simulink model "ModeInt"  (R2018b)
settings: Solver=FixedStepDiscrete  StartTime=0.0  StopTime=10.0  FixedStep=0.01  RelTol=1e-3
undefined symbols (not defined in the file or in its folder): c, CmprtMdHMIReqTp1, e, IfVeSMSeStNumConfig, MdReqTp1
(part 1 of 4)
settings Model: Creator=su3dcu  LastModifiedBy=su3dcu
settings DataIOCC: SaveFormat=StructureWithTime  ReturnWorkspaceOutputs=on
settings OptimizationCC: DefaultParameterBehavior=Inlined  EnhancedBackFolding=on  PassReuseOutputArgsAs=Individual arguments  ZeroExternalMemoryAtStartup=off  ZeroInternalMemoryAtStartup=off  OptimizeBlockOrder=speed  DifferentSizesBufferReuse=on  OptimizationCustomize=off
settings DebuggingCC: ParameterTunabilityLossMsg=error
settings HardwareCC: ProdBitPerPointer=32  ProdBitPerSizeT=32  ProdBitPerPtrDiffT=32  ProdLargestAtomicFloat=None  ProdWordSize=32  ProdHWDeviceType=Renesas->RH850
settings ModelReferenceCC: ModelReferenceNumInstancesAllowed=Single
settings SFSimCC: SimCustomHeaderCode="#include\"Rte_Type.h\""  MATLABDynamicMemAlloc=off
settings RTWCC: SystemTargetFile=autosar.tlc  GenCodeOnly=on  TemplateMakefile=ert_default_tmf  Description=AUTOSAR  GenerateReport=on  IncludeHyperlinkInReport=on  LaunchReport=on  CodeExecutionProfiling=on  GenerateTraceInfo=on  GenerateTraceReport=on  GenerateTraceReportSl=on  GenerateTraceReportSf=on  GenerateTraceReportEml=on  GenerateCodeMetricsReport=on
settings CodeAppCC: ForceParamTrailComments=on  IgnoreCustomStorageClasses=off  MaxIdLength=63  OperatorAnnotations=on  SimulinkDataObjDesc=on  SFDataObjDesc=on  InsertBlockDesc=on
settings STFCustomTargetCC: TargetLangStandard=C99 (ISO)  MultiwordLength=256  ParMdlRefBuildCompliant=on  CompOptLevelCompliant=on  IncludeMdlTerminateFcn=off  CombineOutputUpdateFcns=on  SuppressErrorStatus=on  ERTCustomFileBanners=on  SupportAbsoluteTime=off  PurelyIntegerCode=on  SupportNonFinite=off  SupportComplex=off  SupportContinuousTime=off  SupportNonInlinedSFcns=off  RemoveResetFunc=on  MATLABClassNameForMDSCustomization=Simulink.SoftwareTarget.ERTCustomization  AutosarCompliant=on  UseToolchainInfoCompliant=on  LookupTableObjectStructAxisOrder=2,1,3,4,...  LUTObjectStructOrderEvenSpacing=Size,Table,Breakpoints  SystemTargetFile=autosar.tlc
settings ERTTargetCC: TargetLangStandard=C99 (ISO)  ConcurrentExecutionCompliant=off  IncludeMdlTerminateFcn=off  SuppressErrorStatus=on  SupportAbsoluteTime=off  PurelyIntegerCode=on  SupportNonFinite=off  SupportComplex=off  ModelStepFunctionPrototypeControlCompliant=off  CPPClassGenCompliant=off  AutosarCompliant=on  LookupTableObjectStructAxisOrder=2,1,3,4,...  LUTObjectStructOrderEvenSpacing=Size,Table,Breakpoints  InlinedParameterPlacement=NonHierarchical  ERTCustomFileTemplate=example_file_process.tlc  ERTFilePackagingFormat=Compact
settings ConfigComp: DVTestSuiteOptimization=CombinedObjectives (Nonlinear Extended)  DVDetectActiveLogic=on  DVDetectOutOfBounds=on

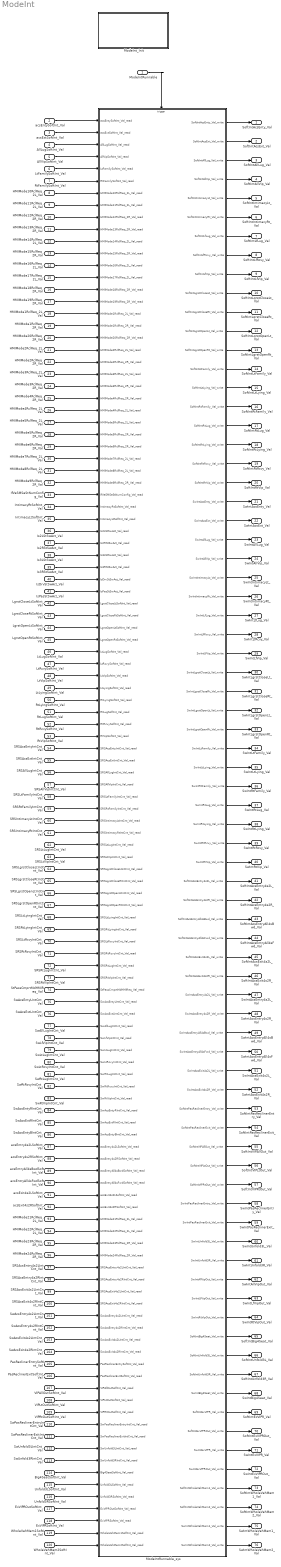
== system ModeInt ==
  ModeIntRunnable : Inport  SampleTime=0.01  OutputFunctionCall=on
  acsEntySoftInt_Val : Inport  Port=2  OutDataTypeStr=IntEnable  PortDimensions=1
  acsExtSoftInt_Val : Inport  Port=3  OutDataTypeStr=IntEnable  PortDimensions=1
  AllLugSoftInt_Val : Inport  Port=4  OutDataTypeStr=IntEnable  PortDimensions=1
  AllVipSoftInt_Val : Inport  Port=5  OutDataTypeStr=IntEnable  PortDimensions=1
  LtFamilySoftInt_Val : Inport  Port=6  OutDataTypeStr=IntEnable  PortDimensions=1
  RtFamilySoftInt_Val : Inport  Port=7  OutDataTypeStr=IntEnable  PortDimensions=1
  HMIMode10RclReq_2L_Val : Inport  Port=8  OutDataTypeStr=Enum: MdReqTp1  PortDimensions=1
  HMIMode11RclReq_2L_Val : Inport  Port=9  OutDataTypeStr=Enum: MdReqTp1  PortDimensions=1
  HMIMode12RclReq_2R_Val : Inport  Port=10  OutDataTypeStr=Enum: MdReqTp1  PortDimensions=1
  HMIMode13RclReq_2R_Val : Inport  Port=11  OutDataTypeStr=Enum: MdReqTp1  PortDimensions=1
  HMIMode14RclReq_2L_Val : Inport  Port=12  OutDataTypeStr=Enum: MdReqTp1  PortDimensions=1
  HMIMode15RclReq_2R_Val : Inport  Port=13  OutDataTypeStr=Enum: MdReqTp1  PortDimensions=1
  HMIMode16RclReq_2L_Val : Inport  Port=14  OutDataTypeStr=Enum: MdReqTp1  PortDimensions=1
  HMIMode17RclReq_2L_Val : Inport  Port=15  OutDataTypeStr=Enum: MdReqTp1  PortDimensions=1
  HMIMode18RclReq_2R_Val : Inport  Port=16  OutDataTypeStr=Enum: MdReqTp1  PortDimensions=1
  HMIMode19RclReq_2R_Val : Inport  Port=17  OutDataTypeStr=Enum: MdReqTp1  PortDimensions=1
  HMIMode1RclReq_2L_Val : Inport  Port=18  OutDataTypeStr=Enum: MdReqTp1  PortDimensions=1
  HMIMode1RclReq_2R_Val : Inport  Port=19  OutDataTypeStr=Enum: MdReqTp1  PortDimensions=1
  HMIMode20RclReq_2R_Val : Inport  Port=20  OutDataTypeStr=Enum: MdReqTp1  PortDimensions=1
  HMIMode2RclReq_2L_Val : Inport  Port=21  OutDataTypeStr=Enum: MdReqTp1  PortDimensions=1
  HMIMode2RclReq_2R_Val : Inport  Port=22  OutDataTypeStr=Enum: MdReqTp1  PortDimensions=1
  HMIMode3RclReq_2L_Val : Inport  Port=23  OutDataTypeStr=Enum: MdReqTp1  PortDimensions=1
  HMIMode3RclReq_2R_Val : Inport  Port=24  OutDataTypeStr=Enum: MdReqTp1  PortDimensions=1
  HMIMode4RclReq_2R_Val : Inport  Port=25  OutDataTypeStr=Enum: MdReqTp1  PortDimensions=1
  HMIMode4RclReq_2L_Val : Inport  Port=26  OutDataTypeStr=Enum: MdReqTp1  PortDimensions=1
  HMIMode5RclReq_2L_Val : Inport  Port=27  OutDataTypeStr=Enum: MdReqTp1  PortDimensions=1
  HMIMode5RclReq_2R_Val : Inport  Port=28  OutDataTypeStr=Enum: MdReqTp1  PortDimensions=1
  HMIMode6RclReq_2R_Val : Inport  Port=29  OutDataTypeStr=Enum: MdReqTp1  PortDimensions=1
  HMIMode7RclReq_2L_Val : Inport  Port=30  OutDataTypeStr=Enum: MdReqTp1  PortDimensions=1
  HMIMode8RclReq_2L_Val : Inport  Port=31  OutDataTypeStr=Enum: MdReqTp1  PortDimensions=1
  HMIMode9RclReq_2R_Val : Inport  Port=32  OutDataTypeStr=Enum: MdReqTp1  PortDimensions=1
  IfVeSMSeStNumConfig_Val : Inport  Port=33  OutDataTypeStr=Enum: IfVeSMSeStNumConfig  PortDimensions=1
  IntimacyRtSoftInt_Val : Inport  Port=34  OutDataTypeStr=IntEnable  PortDimensions=1
  IntimacyLtSoftInt_Val : Inport  Port=35  OutDataTypeStr=IntEnable  PortDimensions=1
  Is2LStSwAct_Val : Inport  Port=36  OutDataTypeStr=boolean  PortDimensions=1
  Is2RStSwAct_Val : Inport  Port=37  OutDataTypeStr=boolean  PortDimensions=1
  Is3LStSwAct_Val : Inport  Port=38  OutDataTypeStr=boolean  PortDimensions=1
  Is3RStSwAct_Val : Inport  Port=39  OutDataTypeStr=boolean  PortDimensions=1
  IsDrvStSwAct_Val : Inport  Port=40  OutDataTypeStr=boolean  PortDimensions=1
  IsPasStSwAct_Val : Inport  Port=41  OutDataTypeStr=boolean  PortDimensions=1
  LgrstCloseLtSoftInt_Val : Inport  Port=42  OutDataTypeStr=IntEnable  PortDimensions=1
  LgrstCloseRtSoftInt_Val : Inport  Port=43  OutDataTypeStr=IntEnable  PortDimensions=1
  LgrstOpenLtSoftInt_Val : Inport  Port=44  OutDataTypeStr=IntEnable  PortDimensions=1
  LgrstOpenRtSoftInt_Val : Inport  Port=45  OutDataTypeStr=IntEnable  PortDimensions=1
  LtLugSoftInt_Val : Inport  Port=46  OutDataTypeStr=IntEnable  PortDimensions=1
  LtRcvySoftInt_Val : Inport  Port=47  OutDataTypeStr=IntEnable  PortDimensions=1
  LtVipSoftInt_Val : Inport  Port=48  OutDataTypeStr=IntEnable  PortDimensions=1
  LtLyingSoftInt_Val : Inport  Port=49  OutDataTypeStr=IntEnable  PortDimensions=1
  RtLyingSoftInt_Val : Inport  Port=50  OutDataTypeStr=IntEnable  PortDimensions=1
  RtLugSoftInt_Val : Inport  Port=51  OutDataTypeStr=IntEnable  PortDimensions=1
  RtRcvySoftInt_Val : Inport  Port=52  OutDataTypeStr=IntEnable  PortDimensions=1
  RtVipSoftInt_Val : Inport  Port=53  OutDataTypeStr=IntEnable  PortDimensions=1
  SRSAcsEntyIntCnt_Val : Inport  Port=54  OutDataTypeStr=IntCnt  PortDimensions=1
  SRSAcsExtIntCnt_Val : Inport  Port=55  OutDataTypeStr=IntCnt  PortDimensions=1
  SRSAllLugIntCnt_Val : Inport  Port=56  OutDataTypeStr=IntCnt  PortDimensions=1
  SRSAllVipIntCnt_Val : Inport  Port=57  OutDataTypeStr=IntCnt  PortDimensions=1
  SRSLtFamilyIntCnt_Val : Inport  Port=58  OutDataTypeStr=IntCnt  PortDimensions=1
  SRSRtFamilyIntCnt_Val : Inport  Port=59  OutDataTypeStr=IntCnt  PortDimensions=1
  SRSIntimacyLtIntCnt_Val : Inport  Port=60  OutDataTypeStr=IntCnt  PortDimensions=1
  SRSIntimacyRtIntCnt_Val : Inport  Port=61  OutDataTypeStr=IntCnt  PortDimensions=1
  SRSLtLugIntCnt_Val : Inport  Port=62  OutDataTypeStr=IntCnt  PortDimensions=1
  SRSLtVipIntCnt_Val : Inport  Port=63  OutDataTypeStr=IntCnt  PortDimensions=1
  SRSLgrstCloseLtIntCnt_Val : Inport  Port=64  OutDataTypeStr=IntCnt  PortDimensions=1
  SRSLgrstCloseRtIntCnt_Val : Inport  Port=65  OutDataTypeStr=IntCnt  PortDimensions=1
  SRSLgrstOpenLtIntCnt_Val : Inport  Port=66  OutDataTypeStr=IntCnt  PortDimensions=1
  SRSLgrstOpenRtIntCnt_Val : Inport  Port=67  OutDataTypeStr=IntCnt  PortDimensions=1
  SRSLtLyingIntCnt_Val : Inport  Port=68  OutDataTypeStr=IntCnt  PortDimensions=1
  SRSRtLyingIntCnt_Val : Inport  Port=69  OutDataTypeStr=IntCnt  PortDimensions=1
  SRSLtRcvyIntCnt_Val : Inport  Port=70  OutDataTypeStr=IntCnt  PortDimensions=1
  SRSRtRcvyIntCnt_Val : Inport  Port=71  OutDataTypeStr=IntCnt  PortDimensions=1
  SRSRtLugIntCnt_Val : Inport  Port=72  OutDataTypeStr=IntCnt  PortDimensions=1
  SRSRtVipIntCnt_Val : Inport  Port=73  OutDataTypeStr=IntCnt  PortDimensions=1
  StPassCmprtMdHMIReq_Val : Inport  Port=74  OutDataTypeStr=Enum: CmprtMdHMIReqTp1  PortDimensions=1
  SwAcsEntyLIntCnt_Val : Inport  Port=75  OutDataTypeStr=IntCnt  PortDimensions=1
  SwAcsExtLIntCnt_Val : Inport  Port=76  OutDataTypeStr=IntCnt  PortDimensions=1
  SwAllLugIntCnt_Val : Inport  Port=77  OutDataTypeStr=IntCnt  PortDimensions=1
  SwLfVipIntCnt_Val : Inport  Port=78  OutDataTypeStr=IntCnt  PortDimensions=1
  SwLtLugIntCnt_Val : Inport  Port=79  OutDataTypeStr=IntCnt  PortDimensions=1
  SwLtRcvyIntCnt_Val : Inport  Port=80  OutDataTypeStr=IntCnt  PortDimensions=1
  SwRtLugIntCnt_Val : Inport  Port=81  OutDataTypeStr=IntCnt  PortDimensions=1
  SwRtRcvyIntCnt_Val : Inport  Port=82  OutDataTypeStr=IntCnt  PortDimensions=1
  SwRtVipIntCnt_Val : Inport  Port=83  OutDataTypeStr=IntCnt  PortDimensions=1
  SwAcsEntyRIntCnt_Val : Inport  Port=84  OutDataTypeStr=IntCnt  PortDimensions=1
  SwAcsExtRIntCnt_Val : Inport  Port=85  OutDataTypeStr=IntCnt  PortDimensions=1
  SwAcsEntyBIntCnt_Val : Inport  Port=86  OutDataTypeStr=IntCnt  PortDimensions=1
  acsEntry4s2LSoftInt_Val : Inport  Port=87  OutDataTypeStr=IntEnable  PortDimensions=1
  acsEntry4s2RSoftInt_Val : Inport  Port=88  OutDataTypeStr=IntEnable  PortDimensions=1
  acsEntryAll4sBwdSoftInt_Val : Inport  Port=89  OutDataTypeStr=IntEnable  PortDimensions=1
  acsEntryAll4sFwdSoftInt_Val : Inport  Port=90  OutDataTypeStr=IntEnable  PortDimensions=1
  acsExit4s2LSoftInt_Val : Inport  Port=91  OutDataTypeStr=IntEnable  PortDimensions=1
  acsExit4s2RSoftInt_Val : Inport  Port=92  OutDataTypeStr=IntEnable  PortDimensions=1
  HMIMode21RclReq_2L_Val : Inport  Port=93  OutDataTypeStr=Enum: MdReqTp1  PortDimensions=1
  HMIMode22RclReq_2L_Val : Inport  Port=94  OutDataTypeStr=Enum: MdReqTp1  PortDimensions=1
  HMIMode23RclReq_2R_Val : Inport  Port=95  OutDataTypeStr=Enum: MdReqTp1  PortDimensions=1
  HMIMode24RclReq_2R_Val : Inport  Port=96  OutDataTypeStr=Enum: MdReqTp1  PortDimensions=1
  SRSAcsEntry4s2LIntCnt_Val : Inport  Port=97  OutDataTypeStr=IntCnt  PortDimensions=1
  SRSAcsEntry4s2RIntCnt_Val : Inport  Port=98  OutDataTypeStr=IntCnt  PortDimensions=1
  SRSAcsExit4s2LIntCnt_Val : Inport  Port=99  OutDataTypeStr=IntCnt  PortDimensions=1
  SRSAcsExit4s2RIntCnt_Val : Inport  Port=100  OutDataTypeStr=IntCnt  PortDimensions=1
  SwAcsEntry4s2LIntCnt_Val : Inport  Port=101  OutDataTypeStr=IntCnt  PortDimensions=1
  SwAcsEntry4s2RIntCnt_Val : Inport  Port=102  OutDataTypeStr=IntCnt  PortDimensions=1
  SwAcsExit4s2LIntCnt_Val : Inport  Port=103  OutDataTypeStr=IntCnt  PortDimensions=1
  SwAcsExit4s2RIntCnt_Val : Inport  Port=104  OutDataTypeStr=IntCnt  PortDimensions=1
  PasReclinerEntrySoftInt_Val : Inport  Port=105  OutDataTypeStr=IntEnable  PortDimensions=1
  PasReclinerExitSoftInt_Val : Inport  Port=106  OutDataTypeStr=IntEnable  PortDimensions=1
  VIPAllOutSoftInt_Val : Inport  Port=107  OutDataTypeStr=IntEnable  PortDimensions=1
  VIPLtOutSoftInt_Val : Inport  Port=108  OutDataTypeStr=IntEnable  PortDimensions=1
  VIPRtOutSoftInt_Val : Inport  Port=109  OutDataTypeStr=IntEnable  PortDimensions=1
  SwPasReclinerEntryIntCnt_Val : Inport  Port=110  OutDataTypeStr=IntCnt  PortDimensions=1
  SwPasReclinerExitIntCnt_Val : Inport  Port=111  OutDataTypeStr=IntCnt  PortDimensions=1
  SwUnfold3LIntCnt_Val : Inport  Port=112  OutDataTypeStr=IntCnt  PortDimensions=1
  SwUnfold3RIntCnt_Val : Inport  Port=113  OutDataTypeStr=IntCnt  PortDimensions=1
  Big4SeatSoftInt_Val : Inport  Port=114  OutDataTypeStr=IntEnable  PortDimensions=1
  Unfold3LSoftInt_Val : Inport  Port=115  OutDataTypeStr=IntEnable  PortDimensions=1
  Unfold3RSoftInt_Val : Inport  Port=116  OutDataTypeStr=IntEnable  PortDimensions=1
  ExVIPROutSoftInt_Val : Inport  Port=117  OutDataTypeStr=IntEnable  PortDimensions=1
  ExVIPRSoftInt_Val : Inport  Port=118  OutDataTypeStr=IntEnable  PortDimensions=1
  WholeVehMem1SoftInt_Val : Inport  Port=119  OutDataTypeStr=IntEnable  PortDimensions=1
  WholeVehMem2SoftInt_Val : Inport  Port=120  OutDataTypeStr=IntEnable  PortDimensions=1
  ModeIntRunnable_sys : Subsystem
  ModeInt_Init : Subsystem
  SoftIntAcsEnty_Val : Outport  OutDataTypeStr=IntEnable  PortDimensions=1
  SoftIntAcsExt_Val : Outport  Port=2  OutDataTypeStr=IntEnable  PortDimensions=1
  SoftIntAllLug_Val : Outport  Port=3  OutDataTypeStr=IntEnable  PortDimensions=1
  SoftIntAllVip_Val : Outport  Port=4  OutDataTypeStr=IntEnable  PortDimensions=1
  SoftIntIntimacyLt_Val : Outport  Port=5  OutDataTypeStr=IntEnable  PortDimensions=1
  SoftIntIntimacyRt_Val : Outport  Port=6  OutDataTypeStr=IntEnable  PortDimensions=1
  SoftIntLfLug_Val : Outport  Port=7  OutDataTypeStr=IntEnable  PortDimensions=1
  SoftIntLfRcvy_Val : Outport  Port=8  OutDataTypeStr=IntEnable  PortDimensions=1
  SoftIntLfVip_Val : Outport  Port=9  OutDataTypeStr=IntEnable  PortDimensions=1
  SoftIntLgrstCloseLt_Val : Outport  Port=10  OutDataTypeStr=IntEnable  PortDimensions=1
  SoftIntLgrstCloseRt_Val : Outport  Port=11  OutDataTypeStr=IntEnable  PortDimensions=1
  SoftIntLgrstOpenLt_Val : Outport  Port=12  OutDataTypeStr=IntEnable  PortDimensions=1
  SoftIntLgrstOpenRt_Val : Outport  Port=13  OutDataTypeStr=IntEnable  PortDimensions=1
  SoftIntLtFamily_Val : Outport  Port=14  OutDataTypeStr=IntEnable  PortDimensions=1
  SoftIntLtLying_Val : Outport  Port=15  OutDataTypeStr=IntEnable  PortDimensions=1
  SoftIntRtFamily_Val : Outport  Port=16  OutDataTypeStr=IntEnable  PortDimensions=1
  SoftIntRtLug_Val : Outport  Port=17  OutDataTypeStr=IntEnable  PortDimensions=1
  SoftIntRtLying_Val : Outport  Port=18  OutDataTypeStr=IntEnable  PortDimensions=1
  SoftIntRtRcvy_Val : Outport  Port=19  OutDataTypeStr=IntEnable  PortDimensions=1
  SoftIntRtVip_Val : Outport  Port=20  OutDataTypeStr=IntEnable  PortDimensions=1
  SwIntAcsEnty_Val : Outport  Port=21  OutDataTypeStr=IntEnable  PortDimensions=1
  SwIntAcsExt_Val : Outport  Port=22  OutDataTypeStr=IntEnable  PortDimensions=1
  SwIntAllLug_Val : Outport  Port=23  OutDataTypeStr=IntEnable  PortDimensions=1
  SwIntAllVip_Val : Outport  Port=24  OutDataTypeStr=IntEnable  PortDimensions=1
  SwIntIntimacyLt_Val : Outport  Port=25  OutDataTypeStr=IntEnable  PortDimensions=1
  SwIntIntimacyRt_Val : Outport  Port=26  OutDataTypeStr=IntEnable  PortDimensions=1
  SwIntLfLug_Val : Outport  Port=27  OutDataTypeStr=IntEnable  PortDimensions=1
  SwIntLfRcvy_Val : Outport  Port=28  OutDataTypeStr=IntEnable  PortDimensions=1
  SwIntLfVip_Val : Outport  Port=29  OutDataTypeStr=IntEnable  PortDimensions=1
  SwIntLgrstCloseLt_Val : Outport  Port=30  OutDataTypeStr=IntEnable  PortDimensions=1
  SwIntLgrstCloseRt_Val : Outport  Port=31  OutDataTypeStr=IntEnable  PortDimensions=1
  SwIntLgrstOpenLt_Val : Outport  Port=32  OutDataTypeStr=IntEnable  PortDimensions=1
  SwIntLgrstOpenRt_Val : Outport  Port=33  OutDataTypeStr=IntEnable  PortDimensions=1
  SwIntLtFamily_Val : Outport  Port=34  OutDataTypeStr=IntEnable  PortDimensions=1
  SwIntLtLying_Val : Outport  Port=35  OutDataTypeStr=IntEnable  PortDimensions=1
  SwIntRtFamily_Val : Outport  Port=36  OutDataTypeStr=IntEnable  PortDimensions=1
  SwIntRtLug_Val : Outport  Port=37  OutDataTypeStr=IntEnable  PortDimensions=1
  SwIntRtLying_Val : Outport  Port=38  OutDataTypeStr=IntEnable  PortDimensions=1
  SwIntRtRcvy_Val : Outport  Port=39  OutDataTypeStr=IntEnable  PortDimensions=1
  SwIntRtVip_Val : Outport  Port=40  OutDataTypeStr=IntEnable  PortDimensions=1
  SoftIntAcsEntry4s2L_Val : Outport  Port=41  OutDataTypeStr=IntEnable  PortDimensions=1
  SoftIntAcsEntry4s2R_Val : Outport  Port=42  OutDataTypeStr=IntEnable  PortDimensions=1
  SoftIntAcsEntryAll4sBwd_Val : Outport  Port=43  OutDataTypeStr=IntEnable  PortDimensions=1
  SoftIntAcsEntryAll4sFwd_Val : Outport  Port=44  OutDataTypeStr=IntEnable  PortDimensions=1
  SoftIntAcsExit4s2L_Val : Outport  Port=45  OutDataTypeStr=IntEnable  PortDimensions=1
  SoftIntAcsExit4s2R_Val : Outport  Port=46  OutDataTypeStr=IntEnable  PortDimensions=1
  SwIntAcsEntry4s2L_Val : Outport  Port=47  OutDataTypeStr=IntEnable  PortDimensions=1
  SwIntAcsEntry4s2R_Val : Outport  Port=48  OutDataTypeStr=IntEnable  PortDimensions=1
  SwIntAcsEntryAll4sBwd_Val : Outport  Port=49  OutDataTypeStr=IntEnable  PortDimensions=1
  SwIntAcsEntryAll4sFwd_Val : Outport  Port=50  OutDataTypeStr=IntEnable  PortDimensions=1
  SwIntAcsExit4s2L_Val : Outport  Port=51  OutDataTypeStr=IntEnable  PortDimensions=1
  SwIntAcsExit4s2R_Val : Outport  Port=52  OutDataTypeStr=IntEnable  PortDimensions=1
  SoftIntPasReclinerEntry_Val : Outport  Port=53  OutDataTypeStr=IntEnable  PortDimensions=1
  SoftIntPasReclinerExit_Val : Outport  Port=54  OutDataTypeStr=IntEnable  PortDimensions=1
  SoftIntVIPAllOut_Val : Outport  Port=55  OutDataTypeStr=IntEnable  PortDimensions=1
  SoftIntVIPLtOut_Val : Outport  Port=56  OutDataTypeStr=IntEnable  PortDimensions=1
  SoftIntVIPRtOut_Val : Outport  Port=57  OutDataTypeStr=IntEnable  PortDimensions=1
  SwIntPasReclinerEntry_Val : Outport  Port=58  OutDataTypeStr=IntEnable  PortDimensions=1
  SwIntPasReclinerExit_Val : Outport  Port=59  OutDataTypeStr=IntEnable  PortDimensions=1
  SwIntUnfold3L_Val : Outport  Port=60  OutDataTypeStr=IntEnable  PortDimensions=1
  SwIntUnfold3R_Val : Outport  Port=61  OutDataTypeStr=IntEnable  PortDimensions=1
  SwIntAllVipOut_Val : Outport  Port=62  OutDataTypeStr=IntEnable  PortDimensions=1
  SwIntLfVipOut_Val : Outport  Port=63  OutDataTypeStr=IntEnable  PortDimensions=1
  SwIntRtVipOut_Val : Outport  Port=64  OutDataTypeStr=IntEnable  PortDimensions=1
  SoftIntBig4Seat_Val : Outport  Port=65  OutDataTypeStr=IntEnable  PortDimensions=1
  SoftIntUnfold3L_Val : Outport  Port=66  OutDataTypeStr=IntEnable  PortDimensions=1
  SoftIntUnfold3R_Val : Outport  Port=67  OutDataTypeStr=IntEnable  PortDimensions=1
  SwIntBig4Seat_Val : Outport  Port=68  OutDataTypeStr=IntEnable  PortDimensions=1
  SoftIntExVIPR_Val : Outport  Port=69  OutDataTypeStr=IntEnable  PortDimensions=1
  SoftIntExVIPROut_Val : Outport  Port=70  OutDataTypeStr=IntEnable  PortDimensions=1
  SwIntExVIPR_Val : Outport  Port=71  OutDataTypeStr=IntEnable  PortDimensions=1
  SwIntExVIPROut_Val : Outport  Port=72  OutDataTypeStr=IntEnable  PortDimensions=1
  SoftIntWholeVehMem1_Val : Outport  Port=73  OutDataTypeStr=IntEnable  PortDimensions=1
  SoftIntWholeVehMem2_Val : Outport  Port=74  OutDataTypeStr=IntEnable  PortDimensions=1
  SwIntWholeVehMem1_Val : Outport  Port=75  OutDataTypeStr=IntEnable  PortDimensions=1
  SwIntWholeVehMem2_Val : Outport  Port=76  OutDataTypeStr=IntEnable  PortDimensions=1
  wires:
  acsEntySoftInt_Val/1 -> ModeIntRunnable_sys/1(acsEntySoftInt_Val_read)
  acsExtSoftInt_Val/1 -> ModeIntRunnable_sys/2(acsExtSoftInt_Val_read)
  AllLugSoftInt_Val/1 -> ModeIntRunnable_sys/3(AllLugSoftInt_Val_read)
  AllVipSoftInt_Val/1 -> ModeIntRunnable_sys/4(AllVipSoftInt_Val_read)
  LtFamilySoftInt_Val/1 -> ModeIntRunnable_sys/5(LtFamilySoftInt_Val_read)
  RtFamilySoftInt_Val/1 -> ModeIntRunnable_sys/6(RtFamilySoftInt_Val_read)
  HMIMode10RclReq_2L_Val/1 -> ModeIntRunnable_sys/7(HMIMode10RclReq_2L_Val_read)
  HMIMode11RclReq_2L_Val/1 -> ModeIntRunnable_sys/8(HMIMode11RclReq_2L_Val_read)
  HMIMode12RclReq_2R_Val/1 -> ModeIntRunnable_sys/9(HMIMode12RclReq_2R_Val_read)
  HMIMode13RclReq_2R_Val/1 -> ModeIntRunnable_sys/10(HMIMode13RclReq_2R_Val_read)
  HMIMode14RclReq_2L_Val/1 -> ModeIntRunnable_sys/11(HMIMode14RclReq_2L_Val_read)
  HMIMode15RclReq_2R_Val/1 -> ModeIntRunnable_sys/12(HMIMode15RclReq_2R_Val_read)
  HMIMode16RclReq_2L_Val/1 -> ModeIntRunnable_sys/13(HMIMode16RclReq_2L_Val_read)
  HMIMode17RclReq_2L_Val/1 -> ModeIntRunnable_sys/14(HMIMode17RclReq_2L_Val_read)
  HMIMode18RclReq_2R_Val/1 -> ModeIntRunnable_sys/15(HMIMode18RclReq_2R_Val_read)
  HMIMode19RclReq_2R_Val/1 -> ModeIntRunnable_sys/16(HMIMode19RclReq_2R_Val_read)
  HMIMode1RclReq_2L_Val/1 -> ModeIntRunnable_sys/17(HMIMode1RclReq_2L_Val_read)
  HMIMode1RclReq_2R_Val/1 -> ModeIntRunnable_sys/18(HMIMode1RclReq_2R_Val_read)
  HMIMode20RclReq_2R_Val/1 -> ModeIntRunnable_sys/19(HMIMode20RclReq_2R_Val_read)
  HMIMode2RclReq_2L_Val/1 -> ModeIntRunnable_sys/20(HMIMode2RclReq_2L_Val_read)
  HMIMode2RclReq_2R_Val/1 -> ModeIntRunnable_sys/21(HMIMode2RclReq_2R_Val_read)
  HMIMode3RclReq_2L_Val/1 -> ModeIntRunnable_sys/22(HMIMode3RclReq_2L_Val_read)
  HMIMode3RclReq_2R_Val/1 -> ModeIntRunnable_sys/23(HMIMode3RclReq_2R_Val_read)
  HMIMode4RclReq_2R_Val/1 -> ModeIntRunnable_sys/24(HMIMode4RclReq_2R_Val_read)
  HMIMode4RclReq_2L_Val/1 -> ModeIntRunnable_sys/25(HMIMode4RclReq_2L_Val_read)
  HMIMode5RclReq_2L_Val/1 -> ModeIntRunnable_sys/26(HMIMode5RclReq_2L_Val_read)
  HMIMode5RclReq_2R_Val/1 -> ModeIntRunnable_sys/27(HMIMode5RclReq_2R_Val_read)
  HMIMode6RclReq_2R_Val/1 -> ModeIntRunnable_sys/28(HMIMode6RclReq_2R_Val_read)
  HMIMode7RclReq_2L_Val/1 -> ModeIntRunnable_sys/29(HMIMode7RclReq_2L_Val_read)
  HMIMode8RclReq_2L_Val/1 -> ModeIntRunnable_sys/30(HMIMode8RclReq_2L_Val_read)
  HMIMode9RclReq_2R_Val/1 -> ModeIntRunnable_sys/31(HMIMode9RclReq_2R_Val_read)
  IfVeSMSeStNumConfig_Val/1 -> ModeIntRunnable_sys/32(IfVeSMSeStNumConfig_Val_read)
  IntimacyRtSoftInt_Val/1 -> ModeIntRunnable_sys/33(IntimacyRtSoftInt_Val_read)
  IntimacyLtSoftInt_Val/1 -> ModeIntRunnable_sys/34(IntimacyLtSoftInt_Val_read)
  Is2LStSwAct_Val/1 -> ModeIntRunnable_sys/35(Is2LStSwAct_Val_read)
  Is2RStSwAct_Val/1 -> ModeIntRunnable_sys/36(Is2RStSwAct_Val_read)
  Is3LStSwAct_Val/1 -> ModeIntRunnable_sys/37(Is3LStSwAct_Val_read)
  Is3RStSwAct_Val/1 -> ModeIntRunnable_sys/38(Is3RStSwAct_Val_read)
  IsDrvStSwAct_Val/1 -> ModeIntRunnable_sys/39(IsDrvStSwAct_Val_read)
  IsPasStSwAct_Val/1 -> ModeIntRunnable_sys/40(IsPasStSwAct_Val_read)
  LgrstCloseLtSoftInt_Val/1 -> ModeIntRunnable_sys/41(LgrstCloseLtSoftInt_Val_read)
  LgrstCloseRtSoftInt_Val/1 -> ModeIntRunnable_sys/42(LgrstCloseRtSoftInt_Val_read)
  LgrstOpenLtSoftInt_Val/1 -> ModeIntRunnable_sys/43(LgrstOpenLtSoftInt_Val_read)
  LgrstOpenRtSoftInt_Val/1 -> ModeIntRunnable_sys/44(LgrstOpenRtSoftInt_Val_read)
  LtLugSoftInt_Val/1 -> ModeIntRunnable_sys/45(LtLugSoftInt_Val_read)
  LtRcvySoftInt_Val/1 -> ModeIntRunnable_sys/46(LtRcvySoftInt_Val_read)
  LtVipSoftInt_Val/1 -> ModeIntRunnable_sys/47(LtVipSoftInt_Val_read)
  LtLyingSoftInt_Val/1 -> ModeIntRunnable_sys/48(LtLyingSoftInt_Val_read)
  RtLyingSoftInt_Val/1 -> ModeIntRunnable_sys/49(RtLyingSoftInt_Val_read)
  RtLugSoftInt_Val/1 -> ModeIntRunnable_sys/50(RtLugSoftInt_Val_read)
  RtRcvySoftInt_Val/1 -> ModeIntRunnable_sys/51(RtRcvySoftInt_Val_read)
  RtVipSoftInt_Val/1 -> ModeIntRunnable_sys/52(RtVipSoftInt_Val_read)
  SRSAcsEntyIntCnt_Val/1 -> ModeIntRunnable_sys/53(SRSAcsEntyIntCnt_Val_read)
  SRSAcsExtIntCnt_Val/1 -> ModeIntRunnable_sys/54(SRSAcsExtIntCnt_Val_read)
  SRSAllLugIntCnt_Val/1 -> ModeIntRunnable_sys/55(SRSAllLugIntCnt_Val_read)
  SRSAllVipIntCnt_Val/1 -> ModeIntRunnable_sys/56(SRSAllVipIntCnt_Val_read)
  SRSLtFamilyIntCnt_Val/1 -> ModeIntRunnable_sys/57(SRSLtFamilyIntCnt_Val_read)
  SRSRtFamilyIntCnt_Val/1 -> ModeIntRunnable_sys/58(SRSRtFamilyIntCnt_Val_read)
  SRSIntimacyLtIntCnt_Val/1 -> ModeIntRunnable_sys/59(SRSIntimacyLtIntCnt_Val_read)
  SRSIntimacyRtIntCnt_Val/1 -> ModeIntRunnable_sys/60(SRSIntimacyRtIntCnt_Val_read)
  SRSLtLugIntCnt_Val/1 -> ModeIntRunnable_sys/61(SRSLtLugIntCnt_Val_read)
  SRSLtVipIntCnt_Val/1 -> ModeIntRunnable_sys/62(SRSLtVipIntCnt_Val_read)
  SRSLgrstCloseLtIntCnt_Val/1 -> ModeIntRunnable_sys/63(SRSLgrstCloseLtIntCnt_Val_read)
  SRSLgrstCloseRtIntCnt_Val/1 -> ModeIntRunnable_sys/64(SRSLgrstCloseRtIntCnt_Val_read)
  SRSLgrstOpenLtIntCnt_Val/1 -> ModeIntRunnable_sys/65(SRSLgrstOpenLtIntCnt_Val_read)
  SRSLgrstOpenRtIntCnt_Val/1 -> ModeIntRunnable_sys/66(SRSLgrstOpenRtIntCnt_Val_read)
  SRSLtLyingIntCnt_Val/1 -> ModeIntRunnable_sys/67(SRSLtLyingIntCnt_Val_read)
  SRSRtLyingIntCnt_Val/1 -> ModeIntRunnable_sys/68(SRSRtLyingIntCnt_Val_read)
  SRSLtRcvyIntCnt_Val/1 -> ModeIntRunnable_sys/69(SRSLtRcvyIntCnt_Val_read)
  SRSRtRcvyIntCnt_Val/1 -> ModeIntRunnable_sys/70(SRSRtRcvyIntCnt_Val_read)
  SRSRtLugIntCnt_Val/1 -> ModeIntRunnable_sys/71(SRSRtLugIntCnt_Val_read)
  SRSRtVipIntCnt_Val/1 -> ModeIntRunnable_sys/72(SRSRtVipIntCnt_Val_read)
  StPassCmprtMdHMIReq_Val/1 -> ModeIntRunnable_sys/73(StPassCmprtMdHMIReq_Val_read)
  SwAcsEntyLIntCnt_Val/1 -> ModeIntRunnable_sys/74(SwAcsEntyLIntCnt_Val_read)
  SwAcsExtLIntCnt_Val/1 -> ModeIntRunnable_sys/75(SwAcsExtLIntCnt_Val_read)
  SwAllLugIntCnt_Val/1 -> ModeIntRunnable_sys/76(SwAllLugIntCnt_Val_read)
  SwLfVipIntCnt_Val/1 -> ModeIntRunnable_sys/77(SwLfVipIntCnt_Val_read)
  SwLtLugIntCnt_Val/1 -> ModeIntRunnable_sys/78(SwLtLugIntCnt_Val_read)
  SwLtRcvyIntCnt_Val/1 -> ModeIntRunnable_sys/79(SwLtRcvyIntCnt_Val_read)
  SwRtLugIntCnt_Val/1 -> ModeIntRunnable_sys/80(SwRtLugIntCnt_Val_read)
  SwRtRcvyIntCnt_Val/1 -> ModeIntRunnable_sys/81(SwRtRcvyIntCnt_Val_read)
  SwRtVipIntCnt_Val/1 -> ModeIntRunnable_sys/82(SwRtVipIntCnt_Val_read)
  ModeIntRunnable_sys/1(SoftIntAcsEnty_Val_write) -> SoftIntAcsEnty_Val/1
  ModeIntRunnable_sys/2(SoftIntAcsExt_Val_write) -> SoftIntAcsExt_Val/1
  ModeIntRunnable_sys/3(SoftIntAllLug_Val_write) -> SoftIntAllLug_Val/1
  ModeIntRunnable_sys/4(SoftIntAllVip_Val_write) -> SoftIntAllVip_Val/1
  ModeIntRunnable_sys/5(SoftIntIntimacyLt_Val_write) -> SoftIntIntimacyLt_Val/1
  ModeIntRunnable_sys/6(SoftIntIntimacyRt_Val_write) -> SoftIntIntimacyRt_Val/1
  ModeIntRunnable_sys/7(SoftIntLfLug_Val_write) -> SoftIntLfLug_Val/1
  ModeIntRunnable_sys/8(SoftIntLfRcvy_Val_write) -> SoftIntLfRcvy_Val/1
  ModeIntRunnable_sys/9(SoftIntLfVip_Val_write) -> SoftIntLfVip_Val/1
  ModeIntRunnable_sys/10(SoftIntLgrstCloseLt_Val_write) -> SoftIntLgrstCloseLt_Val/1
  ModeIntRunnable_sys/11(SoftIntLgrstCloseRt_Val_write) -> SoftIntLgrstCloseRt_Val/1
  ModeIntRunnable_sys/12(SoftIntLgrstOpenLt_Val_write) -> SoftIntLgrstOpenLt_Val/1
  ModeIntRunnable_sys/13(SoftIntLgrstOpenRt_Val_write) -> SoftIntLgrstOpenRt_Val/1
  ModeIntRunnable_sys/14(SoftIntLtFamily_Val_write) -> SoftIntLtFamily_Val/1
  ModeIntRunnable_sys/15(SoftIntLtLying_Val_write) -> SoftIntLtLying_Val/1
  ModeIntRunnable_sys/16(SoftIntRtFamily_Val_write) -> SoftIntRtFamily_Val/1
  ModeIntRunnable_sys/17(SoftIntRtLug_Val_write) -> SoftIntRtLug_Val/1
  ModeIntRunnable_sys/18(SoftIntRtLying_Val_write) -> SoftIntRtLying_Val/1
  ModeIntRunnable_sys/19(SoftIntRtRcvy_Val_write) -> SoftIntRtRcvy_Val/1
  ModeIntRunnable_sys/20(SoftIntRtVip_Val_write) -> SoftIntRtVip_Val/1
  ModeIntRunnable_sys/21(SwIntAcsEnty_Val_write) -> SwIntAcsEnty_Val/1
  ModeIntRunnable_sys/22(SwIntAcsExt_Val_write) -> SwIntAcsExt_Val/1
  ModeIntRunnable_sys/23(SwIntAllLug_Val_write) -> SwIntAllLug_Val/1
  ModeIntRunnable_sys/24(SwIntAllVip_Val_write) -> SwIntAllVip_Val/1
  ModeIntRunnable_sys/25(SwIntIntimacyLt_Val_write) -> SwIntIntimacyLt_Val/1
  ModeIntRunnable_sys/26(SwIntIntimacyRt_Val_write) -> SwIntIntimacyRt_Val/1
  ModeIntRunnable_sys/27(SwIntLfLug_Val_write) -> SwIntLfLug_Val/1
  ModeIntRunnable_sys/28(SwIntLfRcvy_Val_write) -> SwIntLfRcvy_Val/1
  ModeIntRunnable_sys/29(SwIntLfVip_Val_write) -> SwIntLfVip_Val/1
  ModeIntRunnable_sys/30(SwIntLgrstCloseLt_Val_write) -> SwIntLgrstCloseLt_Val/1
  ModeIntRunnable_sys/31(SwIntLgrstCloseRt_Val_write) -> SwIntLgrstCloseRt_Val/1
  ModeIntRunnable_sys/32(SwIntLgrstOpenLt_Val_write) -> SwIntLgrstOpenLt_Val/1
  ModeIntRunnable_sys/33(SwIntLgrstOpenRt_Val_write) -> SwIntLgrstOpenRt_Val/1
  ModeIntRunnable_sys/34(SwIntLtFamily_Val_write) -> SwIntLtFamily_Val/1
  ModeIntRunnable_sys/35(SwIntLtLying_Val_write) -> SwIntLtLying_Val/1
  ModeIntRunnable_sys/36(SwIntRtFamily_Val_write) -> SwIntRtFamily_Val/1
  ModeIntRunnable_sys/37(SwIntRtLug_Val_write) -> SwIntRtLug_Val/1
  ModeIntRunnable_sys/38(SwIntRtLying_Val_write) -> SwIntRtLying_Val/1
  ModeIntRunnable_sys/39(SwIntRtRcvy_Val_write) -> SwIntRtRcvy_Val/1
  ModeIntRunnable_sys/40(SwIntRtVip_Val_write) -> SwIntRtVip_Val/1
  ModeIntRunnable/1 -> ModeIntRunnable_sys/Trigger
  SwAcsEntyRIntCnt_Val/1 -> ModeIntRunnable_sys/83(SwAcsEntyRIntCnt_Val_read)
  SwAcsExtRIntCnt_Val/1 -> ModeIntRunnable_sys/84(SwAcsExtRIntCnt_Val_read)
  SwAcsEntyBIntCnt_Val/1 -> ModeIntRunnable_sys/85(SwAcsEntyBIntCnt_Val_read)
  acsEntry4s2LSoftInt_Val/1 -> ModeIntRunnable_sys/86(acsEntry4s2LSoftInt_Val_read)
  acsEntry4s2RSoftInt_Val/1 -> ModeIntRunnable_sys/87(acsEntry4s2RSoftInt_Val_read)
  acsEntryAll4sBwdSoftInt_Val/1 -> ModeIntRunnable_sys/88(acsEntryAll4sBwdSoftInt_Val_read)
  acsEntryAll4sFwdSoftInt_Val/1 -> ModeIntRunnable_sys/89(acsEntryAll4sFwdSoftInt_Val_read)
  acsExit4s2LSoftInt_Val/1 -> ModeIntRunnable_sys/90(acsExit4s2LSoftInt_Val_read)
  acsExit4s2RSoftInt_Val/1 -> ModeIntRunnable_sys/91(acsExit4s2RSoftInt_Val_read)
  HMIMode21RclReq_2L_Val/1 -> ModeIntRunnable_sys/92(HMIMode21RclReq_2L_Val_read)
  HMIMode22RclReq_2L_Val/1 -> ModeIntRunnable_sys/93(HMIMode22RclReq_2L_Val_read)
  HMIMode23RclReq_2R_Val/1 -> ModeIntRunnable_sys/94(HMIMode23RclReq_2R_Val_read)
  HMIMode24RclReq_2R_Val/1 -> ModeIntRunnable_sys/95(HMIMode24RclReq_2R_Val_read)
  SRSAcsEntry4s2LIntCnt_Val/1 -> ModeIntRunnable_sys/96(SRSAcsEntry4s2LIntCnt_Val_read)
  SRSAcsEntry4s2RIntCnt_Val/1 -> ModeIntRunnable_sys/97(SRSAcsEntry4s2RIntCnt_Val_read)
  SRSAcsExit4s2LIntCnt_Val/1 -> ModeIntRunnable_sys/98(SRSAcsExit4s2LIntCnt_Val_read)
  SRSAcsExit4s2RIntCnt_Val/1 -> ModeIntRunnable_sys/99(SRSAcsExit4s2RIntCnt_Val_read)
  SwAcsEntry4s2LIntCnt_Val/1 -> ModeIntRunnable_sys/100(SwAcsEntry4s2LIntCnt_Val_read)
  SwAcsEntry4s2RIntCnt_Val/1 -> ModeIntRunnable_sys/101(SwAcsEntry4s2RIntCnt_Val_read)
  SwAcsExit4s2LIntCnt_Val/1 -> ModeIntRunnable_sys/102(SwAcsExit4s2LIntCnt_Val_read)
  SwAcsExit4s2RIntCnt_Val/1 -> ModeIntRunnable_sys/103(SwAcsExit4s2RIntCnt_Val_read)
  ModeIntRunnable_sys/41(SoftIntAcsEntry4s2L_Val_write) -> SoftIntAcsEntry4s2L_Val/1
  ModeIntRunnable_sys/42(SoftIntAcsEntry4s2R_Val_write) -> SoftIntAcsEntry4s2R_Val/1
  ModeIntRunnable_sys/43(SoftIntAcsEntryAll4sBwd_Val_write) -> SoftIntAcsEntryAll4sBwd_Val/1
  ModeIntRunnable_sys/44(SoftIntAcsEntryAll4sFwd_Val_write) -> SoftIntAcsEntryAll4sFwd_Val/1
  ModeIntRunnable_sys/45(SoftIntAcsExit4s2L_Val_write) -> SoftIntAcsExit4s2L_Val/1
  ModeIntRunnable_sys/46(SoftIntAcsExit4s2R_Val_write) -> SoftIntAcsExit4s2R_Val/1
  ModeIntRunnable_sys/47(SwIntAcsEntry4s2L_Val_write) -> SwIntAcsEntry4s2L_Val/1
  ModeIntRunnable_sys/48(SwIntAcsEntry4s2R_Val_write) -> SwIntAcsEntry4s2R_Val/1
  ModeIntRunnable_sys/49(SwIntAcsEntryAll4sBwd_Val_write) -> SwIntAcsEntryAll4sBwd_Val/1
  ModeIntRunnable_sys/50(SwIntAcsEntryAll4sFwd_Val_write) -> SwIntAcsEntryAll4sFwd_Val/1
  ModeIntRunnable_sys/51(SwIntAcsExit4s2L_Val_write) -> SwIntAcsExit4s2L_Val/1
  ModeIntRunnable_sys/52(SwIntAcsExit4s2R_Val_write) -> SwIntAcsExit4s2R_Val/1
  PasReclinerEntrySoftInt_Val/1 -> ModeIntRunnable_sys/104(PasReclinerEntrySoftInt_Val_read)
  PasReclinerExitSoftInt_Val/1 -> ModeIntRunnable_sys/105(PasReclinerExitSoftInt_Val_read)
  VIPAllOutSoftInt_Val/1 -> ModeIntRunnable_sys/106(VIPAllOutSoftInt_Val_read)
  VIPLtOutSoftInt_Val/1 -> ModeIntRunnable_sys/107(VIPLtOutSoftInt_Val_read)
  VIPRtOutSoftInt_Val/1 -> ModeIntRunnable_sys/108(VIPRtOutSoftInt_Val_read)
  SwPasReclinerEntryIntCnt_Val/1 -> ModeIntRunnable_sys/109(SwPasReclinerEntryIntCnt_Val_read)
  SwPasReclinerExitIntCnt_Val/1 -> ModeIntRunnable_sys/110(SwPasReclinerExitIntCnt_Val_read)
  SwUnfold3LIntCnt_Val/1 -> ModeIntRunnable_sys/111(SwUnfold3LIntCnt_Val_read)
  SwUnfold3RIntCnt_Val/1 -> ModeIntRunnable_sys/112(SwUnfold3RIntCnt_Val_read)
  ModeIntRunnable_sys/53(SoftIntPasReclinerEntry_Val_write) -> SoftIntPasReclinerEntry_Val/1
  ModeIntRunnable_sys/54(SoftIntPasReclinerExit_Val_write) -> SoftIntPasReclinerExit_Val/1
  ModeIntRunnable_sys/55(SoftIntVIPAllOut_Val_write) -> SoftIntVIPAllOut_Val/1
  ModeIntRunnable_sys/56(SoftIntVIPLtOut_Val_write) -> SoftIntVIPLtOut_Val/1
  ModeIntRunnable_sys/57(SoftIntVIPRtOut_Val_write) -> SoftIntVIPRtOut_Val/1
  ModeIntRunnable_sys/58(SwIntPasReclinerEntry_Val_write) -> SwIntPasReclinerEntry_Val/1
  ModeIntRunnable_sys/59(SwIntPasReclinerExit_Val_write) -> SwIntPasReclinerExit_Val/1
  ModeIntRunnable_sys/60(SwIntUnfold3L_Val_write) -> SwIntUnfold3L_Val/1
  ModeIntRunnable_sys/61(SwIntUnfold3R_Val_write) -> SwIntUnfold3R_Val/1
  ModeIntRunnable_sys/62(SwIntAllVipOut_Val_write) -> SwIntAllVipOut_Val/1
  ModeIntRunnable_sys/63(SwIntLfVipOut_Val_write) -> SwIntLfVipOut_Val/1
  ModeIntRunnable_sys/64(SwIntRtVipOut_Val_write) -> SwIntRtVipOut_Val/1
  Big4SeatSoftInt_Val/1 -> ModeIntRunnable_sys/113(Big4SeatSoftInt_Val_read)
  Unfold3LSoftInt_Val/1 -> ModeIntRunnable_sys/114(Unfold3LSoftInt_Val_read)
  Unfold3RSoftInt_Val/1 -> ModeIntRunnable_sys/115(Unfold3RSoftInt_Val_read)
  ModeIntRunnable_sys/65(SoftIntBig4Seat_Val_write) -> SoftIntBig4Seat_Val/1
  ModeIntRunnable_sys/66(SoftIntUnfold3L_Val_write) -> SoftIntUnfold3L_Val/1
  ModeIntRunnable_sys/67(SoftIntUnfold3R_Val_write) -> SoftIntUnfold3R_Val/1
  ModeIntRunnable_sys/68(SwIntBig4Seat_Val_write) -> SwIntBig4Seat_Val/1
  ExVIPROutSoftInt_Val/1 -> ModeIntRunnable_sys/116(ExVIPROutSoftInt_Val_read)
  ExVIPRSoftInt_Val/1 -> ModeIntRunnable_sys/117(ExVIPRSoftInt_Val_read)
  ModeIntRunnable_sys/69(SoftIntExVIPR_Val_write) -> SoftIntExVIPR_Val/1
  ModeIntRunnable_sys/70(SoftIntExVIPROut_Val_write) -> SoftIntExVIPROut_Val/1
  ModeIntRunnable_sys/71(SwIntExVIPR_Val_write) -> SwIntExVIPR_Val/1
  ModeIntRunnable_sys/72(SwIntExVIPROut_Val_write) -> SwIntExVIPROut_Val/1
  WholeVehMem1SoftInt_Val/1 -> ModeIntRunnable_sys/118(WholeVehMem1SoftInt_Val_read)
  WholeVehMem2SoftInt_Val/1 -> ModeIntRunnable_sys/119(WholeVehMem2SoftInt_Val_read)
  ModeIntRunnable_sys/73(SoftIntWholeVehMem1_Val_write) -> SoftIntWholeVehMem1_Val/1
  ModeIntRunnable_sys/74(SoftIntWholeVehMem2_Val_write) -> SoftIntWholeVehMem2_Val/1
  ModeIntRunnable_sys/75(SwIntWholeVehMem1_Val_write) -> SwIntWholeVehMem1_Val/1
  ModeIntRunnable_sys/76(SwIntWholeVehMem2_Val_write) -> SwIntWholeVehMem2_Val/1
